simulink model "Machine1_FinalProject"  (R2018b)
settings: Solver=VariableStepAuto  StartTime=0.0  StopTime=0.1  RelTol=1e-3
libraries: fl_lib x17, nesl_utility x7, powerlib_meascontrol x2, powerlib x1
settings Model: Creator=Mahdi  LastModifiedBy=Mahdi

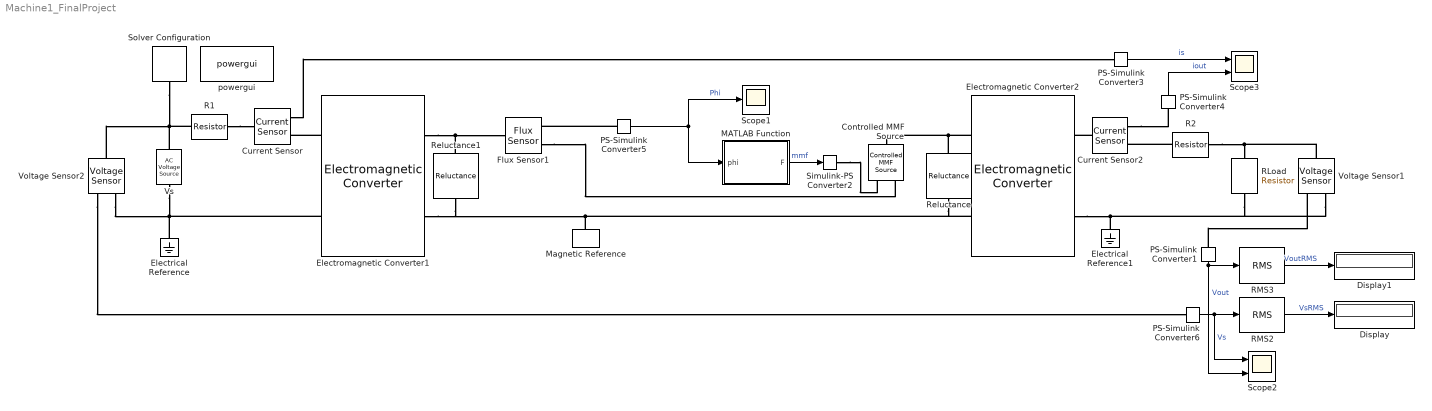
== system Machine1_FinalProject ==
  Controlled MMF Source : fl_lib/Magnetic/Magnetic Sources/Controlled MMF Source
      settings: SourceProductBaseCode=SS
  Current Sensor : fl_lib/Electrical/Electrical Sensors/Current Sensor
  Current Sensor2 : fl_lib/Electrical/Electrical Sensors/Current Sensor
  Display : Display
  Display1 : Display
  Electrical Reference : fl_lib/Electrical/Electrical Elements/Electrical Reference
  Electrical Reference1 : fl_lib/Electrical/Electrical Elements/Electrical Reference
  Electromagnetic Converter1 : fl_lib/Magnetic/Magnetic Elements/Electromagnetic Converter  Nw=230  i_specify=off  i_priority=None  i=0 A  i_nominal_specify=off  i_nominal_unit=A  i_nominal_value=1  v_specify=off  v_priority=None  v=0 V  v_nominal_specify=off  v_nominal_unit=V  v_nominal_value=1  mmf_specify=off  mmf_priority=None  mmf=0 A  mmf_nominal_specify=off  mmf_nominal_unit=A  mmf_nominal_value=1  phi_specify=off  phi_priority=None  phi=0 Wb  phi_nominal_specify=off  phi_nominal_unit=Wb  phi_nominal_value=1
      settings: SourceProductBaseCode=SS
  Electromagnetic Converter2 : fl_lib/Magnetic/Magnetic Elements/Electromagnetic Converter  Nw=40  i_specify=off  i_priority=None  i=0 A  i_nominal_specify=off  i_nominal_unit=A  i_nominal_value=1  v_specify=off  v_priority=None  v=0 V  v_nominal_specify=off  v_nominal_unit=V  v_nominal_value=1  mmf_specify=off  mmf_priority=None  mmf=0 A  mmf_nominal_specify=off  mmf_nominal_unit=A  mmf_nominal_value=1  phi_specify=off  phi_priority=None  phi=0 Wb  phi_nominal_specify=off  phi_nominal_unit=Wb  phi_nominal_value=1
      settings: SourceProductBaseCode=SS
  Flux Sensor1 : fl_lib/Magnetic/Magnetic Sensors/Flux Sensor
      settings: SourceProductName=Simscape  SourceProductBaseCode=SS
  MATLAB Function : MATLAB Function  TreatAsAtomicUnit=on
  Magnetic Reference : fl_lib/Magnetic/Magnetic Elements/Magnetic Reference
      settings: SourceProductName=Simscape  SourceProductBaseCode=SS
  PS-Simulink Converter{1,3..6} (5 alike) : nesl_utility/PS-Simulink Converter  PhysicalDomain=network_engine_domain  SubClassName=ps_output  LeftPortType=input  RightPortType=output  PseudoPeriodic=off  Frequencies=[]  Unit=1  AffineConversion=off
  R1 : fl_lib/Electrical/Electrical Elements/Resistor  R=10 Ohm  i_specify=off  i_priority=None  i=0 A  i_nominal_specify=off  i_nominal_unit=A  i_nominal_value=1  v_specify=off  v_priority=None  v=0 V  v_nominal_specify=off  v_nominal_unit=V  v_nominal_value=1
  R2 : fl_lib/Electrical/Electrical Elements/Resistor  R=0.1 Ohm  i_specify=off  i_priority=None  i=0 A  i_nominal_specify=off  i_nominal_unit=A  i_nominal_value=1  v_specify=off  v_priority=None  v=0 V  v_nominal_specify=off  v_nominal_unit=V  v_nominal_value=1
  RLoad : fl_lib/Electrical/Electrical Elements/Resistor  R=10 Ohm  i_specify=off  i_priority=None  i=0 A  i_nominal_specify=off  i_nominal_unit=A  i_nominal_value=1  v_specify=off  v_priority=None  v=0 V  v_nominal_specify=off  v_nominal_unit=V  v_nominal_value=1
  RMS2 : powerlib_meascontrol/Measurements/RMS  TrueRMS=on  Freq=50  RMSInit=120  Ts=0
  RMS3 : powerlib_meascontrol/Measurements/RMS  TrueRMS=on  Freq=50  RMSInit=120  Ts=0
  Reluctance : fl_lib/Magnetic/Magnetic Elements/Reluctance  g=0.1 m  CSA=0.0625 m^2  mur=1  phi_specify=off  phi_priority=None  phi=0 Wb  phi_nominal_specify=off  phi_nominal_unit=Wb  phi_nominal_value=1  mmf_specify=off  mmf_priority=None  mmf=0 A  mmf_nominal_specify=off  mmf_nominal_unit=A  mmf_nominal_value=1
      settings: SourceProductName=Simscape  SourceProductBaseCode=SS
  Reluctance1 : fl_lib/Magnetic/Magnetic Elements/Reluctance  g=0.1 m  CSA=0.0625 m^2  mur=1  phi_specify=off  phi_priority=None  phi=0 Wb  phi_nominal_specify=off  phi_nominal_unit=Wb  phi_nominal_value=1  mmf_specify=off  mmf_priority=None  mmf=0 A  mmf_nominal_specify=off  mmf_nominal_unit=A  mmf_nominal_value=1
      settings: SourceProductName=Simscape  SourceProductBaseCode=SS
  Scope1 : Scope
  Scope2 : Scope  NumInputPorts=2
  Scope3 : Scope  NumInputPorts=2
  Simulink-PS Converter2 : nesl_utility/Simulink-PS Converter  PhysicalDomain=network_engine_domain  SubClassName=ps_input  LeftPortType=input  RightPortType=output  PseudoPeriodic=off  Frequencies=[]  NoiseDistribution=none  NoiseParameters=[]  Unit=1  AffineConversion=off  FilteringAndDerivatives=provide  SimscapeFilterOrder=1  InputFilterTimeConstant=0.001  UdotUserProvided=0
  Solver Configuration : nesl_utility/Solver Configuration  PhysicalDomain=network_engine_domain  SubClassName=solver  LeftPortType=input  RightPortType=generic  Tones=[]  Harmonics=[]  SimulateNoise=off  Profile=off  UseLocalSampling=off  EnableSwitchedLinearOptims=on  FrequencyDomain=off  UseCCode=off  RelTol=0.001  AbsTol=1e-06  MinStep=1e-09  ToWorkspace=off  RevertToSquareIcSolve=off  NumHomotopyIterations=100  PhasorMode=off  PhasorModeNumHarmonics=1  DoDC=off  ResidualTolerance=1e-09  UseLocalSolver=off  LocalSolverChoice=NE_BACKWARD_EULER_ADVANCER  LocalSolverSampleTime=0.001  DoFixedCost=off  MaxNonlinIter=3  MaxModeIter=2  LinearAlgebra=auto  EquationFormulation=NE_TIME_EF  DelaysMemoryBudget=1024  AutomaticFiltering=on  FilteringTimeConstant=0.001  PartitionStorageMethod=AS_NEEDED  PartitionMemoryBudget=1024
  Voltage Sensor1 : fl_lib/Electrical/Electrical Sensors/Voltage Sensor
  Voltage Sensor2 : fl_lib/Electrical/Electrical Sensors/Voltage Sensor
  Vs : fl_lib/Electrical/Electrical Sources/AC Voltage Source  amp=230*sqrt(2) V  shift=90 deg  frequency=50 Hz  omega=0 rad/s
  powergui : powerlib/powergui  Priority=1  SimulationMode=Continuous  SampleTime=50e-6  frequency=60  Iterations=50  frequencyindice=60  Pbase=100e6  ErrMax=1e-4  UnitsV=kV  UnitsW=MW  buscounter=0  FunctionMessages=off  echomessages=off  EnableUseOfTLC=off  CurrentSourceSwitches=off  DisableSnubberDevices=off  DisableRonSwitches=off  DisableVfSwitches=off  DisplayEquations=off  SolverType=Tustin/Backward Euler (TBE)  Interpol=off  ExternalGateDelay=off  methode=off  Ts=100  x0status=blocks  SPID=on  SwTol=0  HookPort=off  RestoreLinks=warning  ResistiveCurrentMeasurement=off  Frange=[0:2:500]  Ylog=off  Xlog=on  ShowGrid=off  save=off  variable=ZData  structure=0  ZoomFFT=off  StartTime=0.0  cycles=1  DisplayStyle=1  fundamental=60  FreqAxis=off  MaxFrequency=1000  frequencyindicesteady=1  RmsSteady=1  display=off
  wires:
  PS-Simulink Converter3/1 -> Scope3/1  "is"
  PS-Simulink Converter4/1 -> Scope3/2  "iout"
  PS-Simulink Converter5/1 -> Scope1/1, MATLAB Function/1(phi)  "Phi"
  MATLAB Function/1(F) -> Simulink-PS Converter2/1  "mmf"
  PS-Simulink Converter6/1 -> Scope2/1, RMS2/1  "Vs"
  RMS2/1 -> Display/1  "VsRMS"
  PS-Simulink Converter1/1 -> Scope2/2, RMS3/1  "Vout"
  RMS3/1 -> Display1/1  "VoutRMS"
  connections:
  Vs/LConn1 -- Voltage Sensor2/LConn1 -- Solver Configuration/RConn1 -- R1/RConn1
  Flux Sensor1/RConn2 -- Controlled MMF Source/RConn2
  Electrical Reference1/LConn1 -- RLoad/RConn1 -- Voltage Sensor1/RConn2 -- Electromagnetic Converter2/LConn1
  Voltage Sensor1/LConn1 -- R2/LConn1 -- RLoad/LConn1
  Electromagnetic Converter1/LConn2 -- Voltage Sensor2/RConn2 -- Vs/RConn1 -- Electrical Reference/LConn1
  Simulink-PS Converter2/RConn1 -- Controlled MMF Source/RConn1
  Current Sensor2/RConn1 -- PS-Simulink Converter4/LConn1
  Current Sensor/RConn1 -- PS-Simulink Converter3/LConn1
  PS-Simulink Converter5/LConn1 -- Flux Sensor1/RConn1
  Magnetic Reference/LConn1 -- Reluctance/LConn1 -- Electromagnetic Converter2/RConn1 -- Reluctance1/RConn1 -- Electromagnetic Converter1/RConn2
  Current Sensor2/LConn1 -- Electromagnetic Converter2/LConn2
  Electromagnetic Converter2/RConn2 -- Reluctance/RConn1 -- Controlled MMF Source/LConn1
  Electromagnetic Converter1/LConn1 -- Current Sensor/RConn2
  Electromagnetic Converter1/RConn1 -- Reluctance1/LConn1 -- Flux Sensor1/LConn1
  PS-Simulink Converter1/LConn1 -- Voltage Sensor1/RConn1
  Voltage Sensor2/RConn1 -- PS-Simulink Converter6/LConn1
  R2/RConn1 -- Current Sensor2/RConn2
  R1/LConn1 -- Current Sensor/LConn1

== matlab function Machine1_FinalProject/MATLAB Function ==
  data: phi input; F output
function F = fcn(phi)
    A = 0.005;
    Lavg = 0.72;
    B = phi / A;
    H = 0.1431*exp(6.253*B) - 0.1431;
    F = H*Lavg;
end
